simulink model "CH7_3B"  (Simulink 7.5)
settings: Solver=ode45  StartTime=0.0  StopTime=4  RelTol=1e-3
undefined symbols (not defined in the file): Fs, sided, Two
libraries: dspsnks4 x4, dsparch4 x2
settings Model: Creator=xnote  LastModifiedBy=xnote

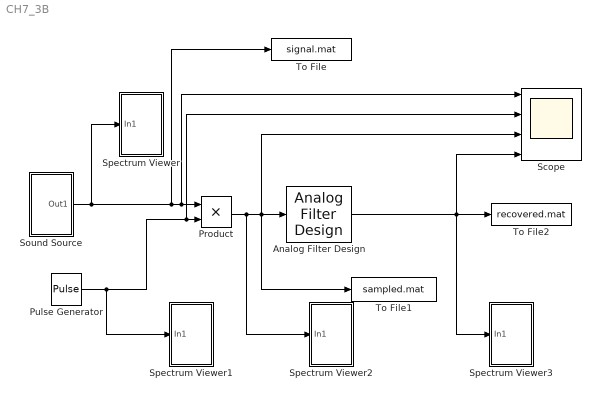
== system CH7_3B ==
  Analog Filter Design : dsparch4/Analog Filter Design  method=Butterworth  filttype=Lowpass  N=8  Wlo=30  Whi=80  Rp=2  Rs=40
  Product : Product  OutDataType=fixdt(1, 16)  OutScaling=2^0  SampleTime=1/(16e4)  RndMeth=Zero
  Pulse Generator : DiscretePulseGenerator  PulseType=Time based  Amplitude=1  Period=10  PulseWidth=5  PhaseDelay=0  SampleTime=1
  Scope : Scope  NumInputPorts=4
      settings: YMin=-0.75~0~-0.75~-0.02  YMax=1~1~0.75~0.1
  Sound Source : Subsystem
  Spectrum Viewer : Subsystem
  Spectrum Viewer1 : Subsystem
  Spectrum Viewer2 : Subsystem
  Spectrum Viewer3 : Subsystem
  To File : ToFile  Filename=signal.mat  SampleTime=1/8192
  To File1 : ToFile  Filename=sampled.mat  SampleTime=1/8192
  To File2 : ToFile  Filename=recovered.mat  SampleTime=1/8192
  wires:
  Sound Source/1(Out1) -> Spectrum Viewer/1(In1), To File/1, Product/1, Scope/1
  Pulse Generator/1 -> Spectrum Viewer1/1(In1), Product/2, Scope/2
  Product/1 -> Spectrum Viewer2/1(In1), Analog Filter Design/1, To File1/1, Scope/3
  Analog Filter Design/1 -> To File2/1, Spectrum Viewer3/1(In1), Scope/4

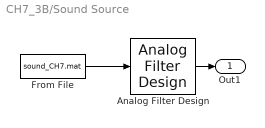
== system CH7_3B/Sound Source ==
  Analog Filter Design : dsparch4/Analog Filter Design  method=Butterworth  filttype=Lowpass  N=8  Wlo=2*pi*4e3  Whi=80  Rp=2  Rs=40
  From File : FromFile  FileName=sound_CH7.mat  SampleTime=0
  Out1 : Outport
  wires:
  From File/1 -> Analog Filter Design/1
  Analog Filter Design/1 -> Out1/1

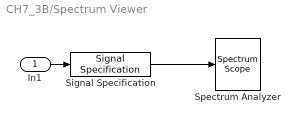
== system CH7_3B/Spectrum Viewer ==
  In1 : Inport
  Signal Specification : SignalSpecification  SampleTime=1/16e4
  Spectrum Analyzer : dspsnks4/Spectrum Scope  DialogController=dspdialog.SpectrumScope  DialogControllerArgs=DataTag0  SystemSampleTime=-1  ScopeProperties=on  Domain=Frequency  HorizSpan=1  UseBuffer=on  BufferSize=1024  Overlap=64  inpFftLenInherit=on  FFTlength=1024  numAvg=200  DisplayProperties=off  AxisGrid=on  Memory=off  FrameNumber=on  AxisLegend=off  AxisZoom=off  OpenScopeAtSimStart=on  OpenScopeImmediately=off  FigPos="[549  354  800  160]"  AxisProperties=off  XUnits=Hertz  XRange=Two-sided ((-Fs/2...Fs/2])  XDisplay=0  InheritXIncr=on  XIncr=1.0  XLabel=Samples  XLimit=Auto  YUnits=dBm  XMax=1  XMin=0  YLabel=Magnitude-squared, dB  LineProperties=off  wintypeSpecScope=Hann  RsSpecScope=50  betaSpecScope=5  winsampSpecScope=Symmetric  XAxisParamsVer=6.9
      settings: YMin=-40  YMax=25
  wires:
  Signal Specification/1 -> Spectrum Analyzer/1
  In1/1 -> Signal Specification/1

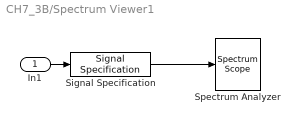
== system CH7_3B/Spectrum Viewer1 ==
  In1 : Inport
  Signal Specification : SignalSpecification  SampleTime=1/16e4
  Spectrum Analyzer : dspsnks4/Spectrum Scope  DialogController=dspdialog.SpectrumScope  DialogControllerArgs=DataTag1  SystemSampleTime=-1  ScopeProperties=on  Domain=Frequency  HorizSpan=1  UseBuffer=on  BufferSize=1024  Overlap=64  inpFftLenInherit=on  FFTlength=1024  numAvg=200  DisplayProperties=off  AxisGrid=on  Memory=off  FrameNumber=on  AxisLegend=off  AxisZoom=off  OpenScopeAtSimStart=on  OpenScopeImmediately=off  FigPos="[549  354  800  160]"  AxisProperties=off  XUnits=Hertz  XRange=Two-sided ((-Fs/2...Fs/2])  XDisplay=0  InheritXIncr=on  XIncr=1.0  XLabel=Samples  XLimit=Auto  YUnits=dBm  XMax=1  XMin=0  YLabel=Magnitude-squared, dB  LineProperties=off  wintypeSpecScope=Hann  RsSpecScope=50  betaSpecScope=5  winsampSpecScope=Symmetric  XAxisParamsVer=6.9
      settings: YMin=-40  YMax=25
  wires:
  In1/1 -> Signal Specification/1
  Signal Specification/1 -> Spectrum Analyzer/1

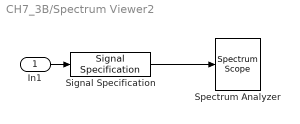
== system CH7_3B/Spectrum Viewer2 ==
  In1 : Inport
  Signal Specification : SignalSpecification  SampleTime=1/16e4
  Spectrum Analyzer : dspsnks4/Spectrum Scope  DialogController=dspdialog.SpectrumScope  DialogControllerArgs=DataTag2  SystemSampleTime=-1  ScopeProperties=on  Domain=Frequency  HorizSpan=1  UseBuffer=on  BufferSize=1024  Overlap=64  inpFftLenInherit=on  FFTlength=1024  numAvg=200  DisplayProperties=off  AxisGrid=on  Memory=off  FrameNumber=on  AxisLegend=off  AxisZoom=off  OpenScopeAtSimStart=on  OpenScopeImmediately=off  FigPos="[549  354  800  160]"  AxisProperties=off  XUnits=Hertz  XRange=Two-sided ((-Fs/2...Fs/2])  XDisplay=0  InheritXIncr=on  XIncr=1.0  XLabel=Samples  XLimit=Auto  YUnits=dBm  XMax=1  XMin=0  YLabel=Magnitude-squared, dB  LineProperties=off  wintypeSpecScope=Hann  RsSpecScope=50  betaSpecScope=5  winsampSpecScope=Symmetric  XAxisParamsVer=6.9
      settings: YMin=-40  YMax=25
  wires:
  Signal Specification/1 -> Spectrum Analyzer/1
  In1/1 -> Signal Specification/1

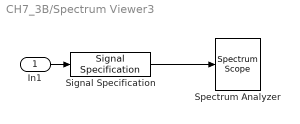
== system CH7_3B/Spectrum Viewer3 ==
  In1 : Inport
  Signal Specification : SignalSpecification  SampleTime=1/16e4
  Spectrum Analyzer : dspsnks4/Spectrum Scope  DialogController=dspdialog.SpectrumScope  DialogControllerArgs=DataTag3  SystemSampleTime=-1  ScopeProperties=on  Domain=Frequency  HorizSpan=1  UseBuffer=on  BufferSize=1024  Overlap=64  inpFftLenInherit=on  FFTlength=1024  numAvg=200  DisplayProperties=off  AxisGrid=on  Memory=off  FrameNumber=on  AxisLegend=off  AxisZoom=off  OpenScopeAtSimStart=on  OpenScopeImmediately=off  FigPos="[549  354  800  160]"  AxisProperties=off  XUnits=Hertz  XRange=Two-sided ((-Fs/2...Fs/2])  XDisplay=0  InheritXIncr=on  XIncr=1.0  XLabel=Samples  XLimit=Auto  YUnits=dBm  XMax=1  XMin=0  YLabel=Magnitude-squared, dB  LineProperties=off  wintypeSpecScope=Hann  RsSpecScope=50  betaSpecScope=5  winsampSpecScope=Symmetric  XAxisParamsVer=6.9
      settings: YMin=-40  YMax=25
  wires:
  In1/1 -> Signal Specification/1
  Signal Specification/1 -> Spectrum Analyzer/1
